simulink model "HighwayLaneChangePlannerTestBench"  (R2024b)
settings: Solver=FixedStepAuto  StartTime=0.0  StopTime=scenario.StopTime  FixedStep=Ts  RelTol=1e-3
PostLoadFcn:
  | helperSLHighwayLaneChangePlannerSetup
values from neighbouring files (symbols this model uses):
  change_difficulty_coeff = 1.0    (= 1)    [helperSLHighwayLaneChangePlannerSetup.m]
  degree = 5    [HelperLCPlannerDefaultData.m]    (also in helperSLHighwayLaneChangePlannerSetup.m)
  egoInitialPose = evalin('base','egoInitialPose')    [HelperPlotLCPlannerStatus.m]    (also in helperSLHighwayLaneChangePlannerSetup.m = struct('ActorID', EgoActor.ActorID,                         )
  lane_change_coeff = 1.0    (= 1)    [helperSLHighwayLaneChangePlannerSetup.m]
  lane_keeping_coeff = 1.0    (= 1)    [helperSLHighwayLaneChangePlannerSetup.m]
  lane_width_coeff = 0.25    [helperSLHighwayLaneChangePlannerSetup.m]
  mapInfo = struct('NumLanes', numLanes,'LaneWidth', zeros(maxNumLanes,1),                  'LaneCenters', zeros(maxNumLanes,1),'NumGlobalPlanPoints',                  size(globalPlanPoints,1), 'GlobalPlanPoints',                  zeros(maxGlobalPlanPoints,2), 'LaneLateralBoundary', zeros(maxNumLanes, 2))    [helperSLHighwayLaneChangePlannerSetup.m]
  MaxFront = 20    [helperSLHighwayLaneChangePlannerSetup.m]
  MaxRear = 20    [helperSLHighwayLaneChangePlannerSetup.m]
  MaxTTC = 5    [helperSLHighwayLaneChangePlannerSetup.m]
  MinTTC = 3    [helperSLHighwayLaneChangePlannerSetup.m]
  num_piece = timeHorizon / 0.5    (= 8)    [helperSLHighwayLaneChangePlannerSetup.m]
  planningResolution = 0.5    [helperSLHighwayLaneChangePlannerSetup.m]
  timeHorizon = 4    [helperSLHighwayLaneChangePlannerSetup.m]
  timeResolution = 0.1    [helperSLHighwayLaneChangePlannerSetup.m]
  Useresample = true    [helperSLHighwayLaneChangePlannerSetup.m]
undefined symbols (not defined in the file or in its folder): actorProfiles, assessment, egoActorID, Feasible_coeff, maxLatAccel, maxLatVelocity, maxLonAccel, maxLonVelocity, minLatVelocity, minLonVelocity, Ts
libraries: simulink x7, drivingscenarioandsensors x2
settings Model: Creator=The MathWorks, Inc.  LastModifiedBy=grape4314
settings SolverCC: ZeroCrossAlgorithm=Adaptive  AlgebraicLoopSolver=TrustRegion  MaxZcPerStep=1
settings DataIOCC: SaveOutput=off  ReturnWorkspaceOutputs=off
settings OptimizationCC: ReuseModelBlockBuffer=off  ZeroExternalMemoryAtStartup=off  ZeroInternalMemoryAtStartup=off  OptimizeBlockOrder=speed
settings DebuggingCC: MaskedZcDiagnostic=none  IgnoredZcDiagnostic=none  UnconnectedInputMsg=warning  UnconnectedOutputMsg=warning  UnconnectedLineMsg=warning  SubsystemReferenceDiagnosticForUnitTest=warning
settings ModelReferenceCC: EnableRefExpFcnMdlSchedulingChecks=on
settings RTWCC: Description=Embedded Coder  SystemTargetFile=ert.tlc  TemplateMakefile=ert_default_tmf  PortableWordSizes=on  CodeProfilingSaveOptions=AllData  TargetLang=C++  GPUComputeCapability=3.5  DLArmComputeVersion=19.05
settings CodeAppCC: ForceParamTrailComments=on  IgnoreCustomStorageClasses=off  OperatorAnnotations=on  SimulinkDataObjDesc=on  SFDataObjDesc=on  InsertBlockDesc=on
settings ERTTargetCC: TargetLangStandard=C++03 (ISO)  GenerateSampleERTMain=on  CodeInterfacePackaging=C++ class  InlinedParameterPlacement=Hierarchical  RootIOFormat=Structure reference  ERTCustomFileTemplate=example_file_process.tlc  DynamicArrayContainerType=coder::array
settings ConfigComp: CovScope=ReferencedModels  CovIncludeTopModel=off  CovMetricSettings=dtrzoibwe

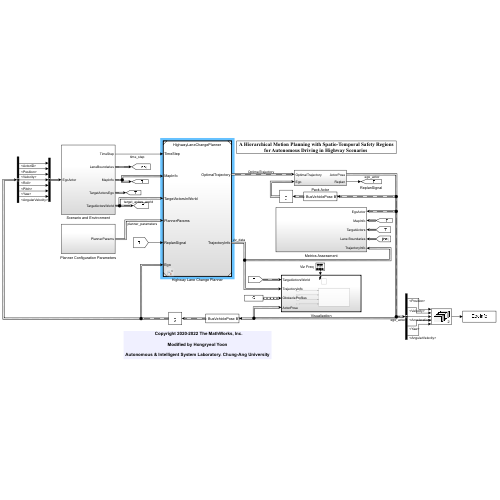
[thumbnail: Simulink's stored preview of the top-level diagram]
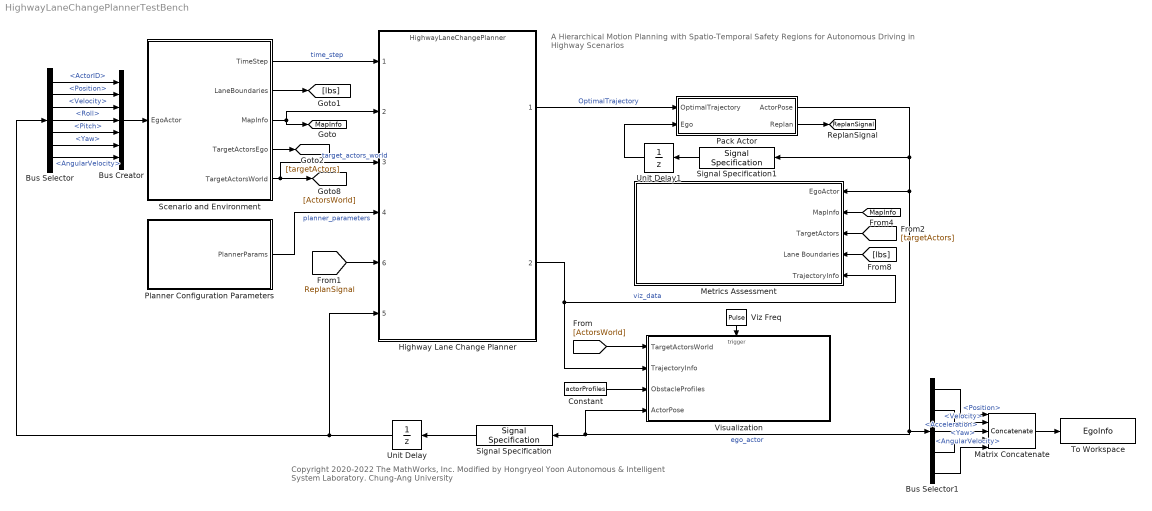
== system HighwayLaneChangePlannerTestBench ==
  note: A Hierarchical Motion Planning with Spatio-Temporal Safety Regions for Autonomous Driving in Highway Scenarios
  note: Copyright 2020-2022 The MathWorks, Inc.
      |
      | Modified by Hongryeol Yoon
      |
      | Autonomous & Intelligent System Laboratory. Chung-Ang University
  Bus Creator : BusCreator  Inputs=7  OutDataTypeStr=Bus: BusVehiclePoseNoAccel
  Bus Selector : BusSelector  OutputSignals=ActorID,Position,Velocity,Roll,Pitch,Yaw,AngularVelocity
  Bus Selector1 : BusSelector  OutputSignals=Position,Velocity,Acceleration,Yaw,AngularVelocity
  Constant : Constant  Value=actorProfiles  OutDataTypeStr=Bus: BusActorProfiles
  Highway Lane Change Planner : ModelReference  ModelNameDialog=HighwayLaneChangePlanner.slx  SimulationMode=Normal  ModelReferenceVersion=10.890
      settings: PortSchema="{\"entries\":[{\"content\":{\"sides\":[{\"content\":{\"connectorIds\":[\"In1\",\"In2\",\"In3\",\"In4\",\"In6\",\"In5\"]},\"type\":\"ConnectorPlacement.EquallySpacedRectSide\",\"uuid\":\"8044d8bb-367a-43f8-b195-4991807fb404\"},{\"content\":{\"connectorIds\":[\"Out1\",\"Out2\"],\"side\":\"RIGHT\"},\"type\":\"ConnectorPlacement.EquallySpacedRectSide\",\"uuid\":\"ee3faf87-dd00-4278-a4db-064b7bf25d12\"},{\"content\":{\"side\":\"TOP\"},\"type\":\"ConnectorPlacement.EquallySpacedRectSide\",\"uuid\":\"9b87e704-685c-45b5-ad58-dd02a7899d78\"}]},\"type\":\"ConnectorPlacement.EquallySpacedConnector\",\"uuid\":\"dfca5ff9-33c4-4b77-827b-e14b0071599c\"}],\"packageUris\":[\"http://schema.mathworks.com/mf0/Connector/R2020b\"],\"version\":\"1.0\"}"
  Matrix Concatenate : Concatenate  NumInputs=5  Mode=Multidimensional array  ConcatenateDimension=2
  Metrics Assessment : Subsystem
  Pack Actor : Subsystem
  Planner Configuration Parameters : Subsystem
  Scenario and Environment : Subsystem
  Signal Specification : SignalSpecification  OutDataTypeStr=Bus: BusVehiclePose  BusOutputAsStruct=on
  Signal Specification1 : SignalSpecification  OutDataTypeStr=Bus: BusVehiclePose  BusOutputAsStruct=on
  To Workspace : ToWorkspace  VariableName=EgoInfo  SaveFormat=Structure With Time  SampleTime=-1
  Unit Delay : UnitDelay  InitialCondition=egoInitialPose  SampleTime=-1  HasFrameUpgradeWarning=on
  Unit Delay1 : UnitDelay  InitialCondition=egoInitialPose  SampleTime=-1  HasFrameUpgradeWarning=on
  Visualization : Subsystem
  Viz Freq : DiscretePulseGenerator  SampleTime=Ts
  tag scope: MapInfo=global, ReplanSignal=global
  wires:
  Scenario and Environment/4(TargetActorsEgo) -> [targetActors]
  Scenario and Environment/2(LaneBoundaries) -> [lbs]
  Highway Lane Change Planner/1 -> Pack Actor/1(OptimalTrajectory)  "OptimalTrajectory"
  Unit Delay/1 -> Bus Selector/1, Highway Lane Change Planner/5
  Signal Specification/1 -> Unit Delay/1
  Scenario and Environment/5(TargetActorsWorld) -> Highway Lane Change Planner/3, [ActorsWorld]  "target_actors_world"
  Scenario and Environment/3(MapInfo) -> Highway Lane Change Planner/2, [MapInfo]
  Constant/1 -> Visualization/3(ObstacleProfiles)
  [ActorsWorld] -> Visualization/1(TargetActorsWorld)
  Planner Configuration Parameters/1(PlannerParams) -> Highway Lane Change Planner/4  "planner_parameters"
  Pack Actor/1(ActorPose) -> Signal Specification1/1, Metrics Assessment/1(EgoActor), Visualization/4(ActorPose), Signal Specification/1, Bus Selector1/1  "ego_actor"
  Highway Lane Change Planner/2 -> Visualization/2(TrajectoryInfo), Metrics Assessment/5(TrajectoryInfo)  "viz_data"
  Scenario and Environment/1(TimeStep) -> Highway Lane Change Planner/1  "time_step"
  [targetActors] -> Metrics Assessment/3(TargetActors)
  [lbs] -> Metrics Assessment/4(Lane Boundaries)
  [MapInfo] -> Metrics Assessment/2(MapInfo)
  Bus Selector/1 -> Bus Creator/1  "<ActorID>"
  Bus Selector/2 -> Bus Creator/2  "<Position>"
  Bus Selector/4 -> Bus Creator/4  "<Roll>"
  Bus Selector/6 -> Bus Creator/6  "<Yaw>"
  Bus Creator/1 -> Scenario and Environment/1(EgoActor)
  Bus Selector/5 -> Bus Creator/5  "<Pitch>"
  Bus Selector/3 -> Bus Creator/3  "<Velocity>"
  Bus Selector/7 -> Bus Creator/7  "<AngularVelocity>"
  Signal Specification1/1 -> Unit Delay1/1
  Unit Delay1/1 -> Pack Actor/2(Ego)
  Pack Actor/2(Replan) -> [ReplanSignal]
  [ReplanSignal] -> Highway Lane Change Planner/6
  Viz Freq/1 -> Visualization/Trigger
  Matrix Concatenate/1 -> To Workspace/1
  Bus Selector1/1 -> Matrix Concatenate/1  "<Position>"
  Bus Selector1/2 -> Matrix Concatenate/2  "<Velocity>"
  Bus Selector1/3 -> Matrix Concatenate/3  "<Acceleration>"
  Bus Selector1/4 -> Matrix Concatenate/4  "<Yaw>"
  Bus Selector1/5 -> Matrix Concatenate/5  "<AngularVelocity>"

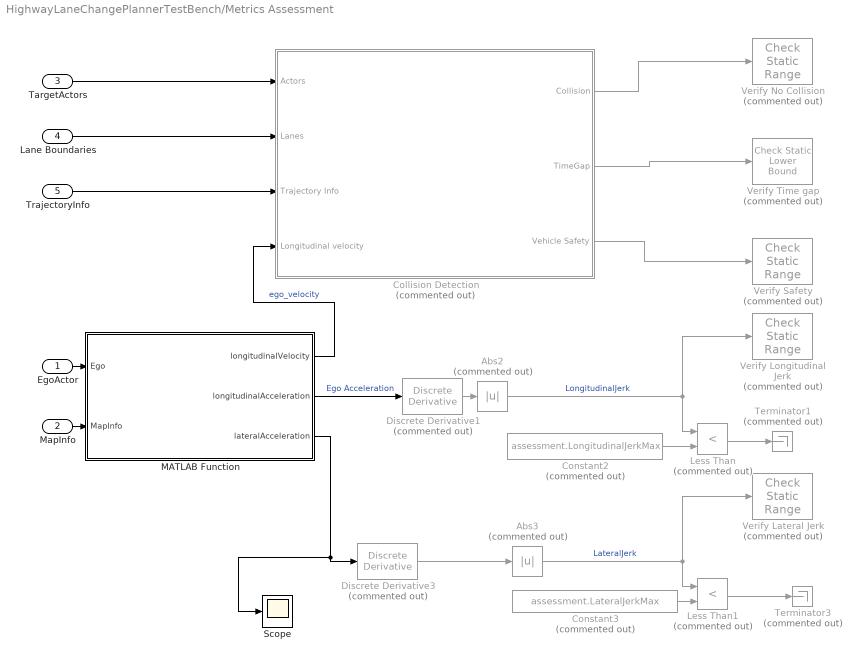
== system HighwayLaneChangePlannerTestBench/Metrics Assessment ==
  EgoActor : Inport
  MapInfo : Inport  Port=2
  TargetActors : Inport  Port=3
  Lane Boundaries : Inport  Port=4
  TrajectoryInfo : Inport  Port=5
  Abs2 : Abs  Commented=on  ZeroCross=off  SaturateOnIntegerOverflow=off
  Abs3 : Abs  Commented=on  ZeroCross=off  SaturateOnIntegerOverflow=off
  Collision Detection : Subsystem  Commented=on
  Constant2 : Constant  Commented=on  Value=assessment.LongitudinalJerkMax
  Constant3 : Constant  Commented=on  Value=assessment.LateralJerkMax
  Discrete Derivative1 : simulink/Discrete/Discrete Derivative  Commented=on  gainval=0.1  ICPrevScaledInput=0.1/Ts  OutMin=[]  OutMax=[]  OutDataType=fixdt(1, 16)  OutScaling=2^-10  DoSatur=off
  Discrete Derivative3 : simulink/Discrete/Discrete Derivative  Commented=on  gainval=0.1  ICPrevScaledInput=0.1/Ts  OutMin=[]  OutMax=[]  OutDataType=fixdt(1, 16)  OutScaling=2^-10  DoSatur=off
  Less Than : RelationalOperator  Commented=on  Operator=<  OutDataTypeStr=boolean  RndMeth=Simplest  InputSameDT=off
  Less Than1 : RelationalOperator  Commented=on  Operator=<  OutDataTypeStr=boolean  RndMeth=Simplest  InputSameDT=off
  MATLAB Function : MATLAB Function  TreatAsAtomicUnit=on
  Scope : Scope
  Terminator1 : Terminator  Commented=on
  Terminator3 : Terminator  Commented=on
  Verify Lateral Jerk : simulink/Model Verification/Check  Static Range  Description=-assessment.LateralJerkMax <= u <= assessment.LateralJerkMax  Commented=on  max=assessment.LateralJerkMax  max_included=on  min=-assessment.LateralJerkMax  min_included=on  enabled=on  stopWhenAssertionFail=off  export=off  icon=graphic
      settings: AttributesFormatString=|
      | ---------------------------------------
      | max = %<max>
      | min = %<min>
  Verify Longitudinal Jerk : simulink/Model Verification/Check  Static Range  Description=-assessment.LongitudinalJerkMax <= u <= assessment.LongitudinalJerkMax  Commented=on  max=assessment.LongitudinalJerkMax  max_included=on  min=-assessment.LongitudinalJerkMax  min_included=on  enabled=on  stopWhenAssertionFail=off  export=off  icon=graphic
      settings: AttributesFormatString=|
      | ---------------------------------------
      | max = %<max>
      | min = %<min>
  Verify No Collision : simulink/Model Verification/Check  Static Range  Description=0 <= u <= 0  Commented=on  max=0  max_included=on  min=0  min_included=on  enabled=on  stopWhenAssertionFail=on  export=off  icon=graphic
  Verify Safety : simulink/Model Verification/Check  Static Range  Description=1 <= u <= 1  Commented=on  max=1  max_included=on  min=1  min_included=on  enabled=on  stopWhenAssertionFail=off  export=off  icon=graphic
  Verify Time gap : simulink/Model Verification/Check Static  Lower Bound  Description=assessment.TimeGap <= u  Commented=on  min=assessment.TimeGap  min_included=on  enabled=on  stopWhenAssertionFail=off  export=off  icon=graphic
      settings: AttributesFormatString=|
      | ---------------------------------------
      | min = %<min>
  wires:
  Collision Detection/1(Collision) -> Verify No Collision/1
  Collision Detection/2(TimeGap) -> Verify Time gap/1
  TrajectoryInfo/1 -> Collision Detection/3(Trajectory Info)
  TargetActors/1 -> Collision Detection/1(Actors)
  Collision Detection/3(Vehicle Safety) -> Verify Safety/1
  Lane Boundaries/1 -> Collision Detection/2(Lanes)
  Discrete Derivative1/1 -> Abs2/1
  Discrete Derivative3/1 -> Abs3/1
  Constant3/1 -> Less Than1/2
  Less Than1/1 -> Terminator3/1
  Constant2/1 -> Less Than/2
  Abs2/1 -> Less Than/1, Verify Longitudinal Jerk/1  "LongitudinalJerk"
  Abs3/1 -> Verify Lateral Jerk/1, Less Than1/1  "LateralJerk"
  Less Than/1 -> Terminator1/1
  EgoActor/1 -> MATLAB Function/1(Ego)
  MapInfo/1 -> MATLAB Function/2(MapInfo)
  MATLAB Function/1(longitudinalVelocity) -> Collision Detection/4(Longitudinal velocity)  "ego_velocity"
  MATLAB Function/2(longitudinalAcceleration) -> Discrete Derivative1/1  "Ego Acceleration"
  MATLAB Function/3(lateralAcceleration) -> Scope/1, Discrete Derivative3/1

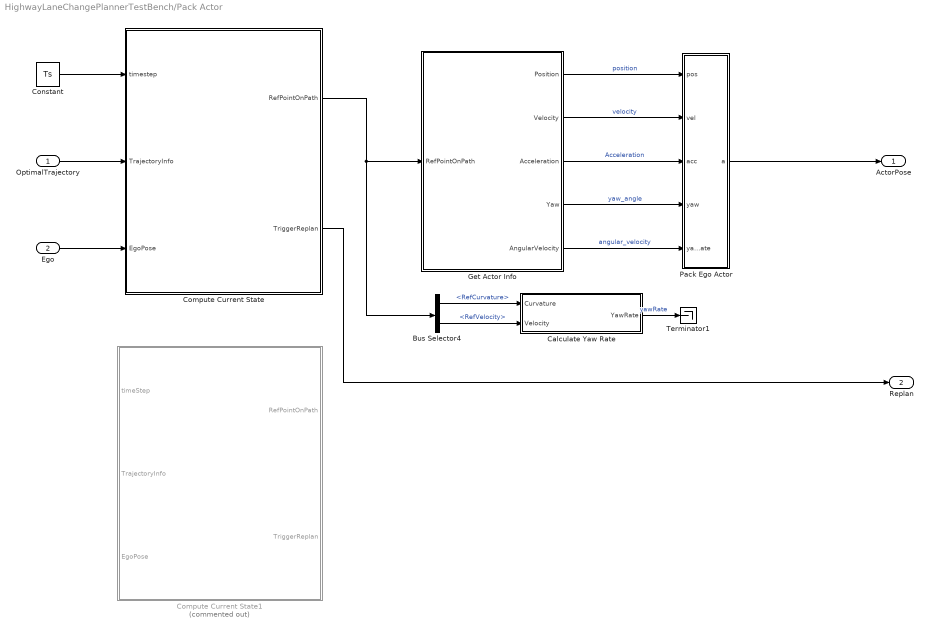
== system HighwayLaneChangePlannerTestBench/Pack Actor ==
  OptimalTrajectory : Inport  SampleTime=Ts
  Ego : Inport  Port=2  OutDataTypeStr=Bus: BusVehiclePose
  Bus Selector4 : BusSelector  OutputSignals=RefCurvature,RefVelocity
  Calculate Yaw Rate : MATLAB Function  TreatAsAtomicUnit=on
  Compute Current State : MATLAB Function  TreatAsAtomicUnit=on
  Compute Current State1 : MATLAB Function  Commented=on  TreatAsAtomicUnit=on
  Constant : Constant  Value=Ts
  Get Actor Info : MATLAB Function  TreatAsAtomicUnit=on
  Pack Ego Actor : MATLAB Function  TreatAsAtomicUnit=on  mask{egoActorID=egoActorID}
      mask prompts: egoActorID "Ego Actor ID"
  Terminator1 : Terminator
  ActorPose : Outport  OutDataTypeStr=Bus: BusVehiclePose
  Replan : Outport  Port=2
  wires:
  Bus Selector4/1 -> Calculate Yaw Rate/1(Curvature)  "<RefCurvature>"
  Bus Selector4/2 -> Calculate Yaw Rate/2(Velocity)  "<RefVelocity>"
  Calculate Yaw Rate/1(YawRate) -> Terminator1/1  "yawRate"
  Pack Ego Actor/1(a) -> ActorPose/1
  Get Actor Info/1(Position) -> Pack Ego Actor/1(pos)  "position"
  Get Actor Info/2(Velocity) -> Pack Ego Actor/2(vel)  "velocity"
  Get Actor Info/3(Acceleration) -> Pack Ego Actor/3(acc)  "Acceleration"
  Get Actor Info/4(Yaw) -> Pack Ego Actor/4(yaw)  "yaw_angle"
  Get Actor Info/5(AngularVelocity) -> Pack Ego Actor/5(yawRate)  "angular_velocity"
  OptimalTrajectory/1 -> Compute Current State/2(TrajectoryInfo)
  Constant/1 -> Compute Current State/1(timestep)
  Ego/1 -> Compute Current State/3(EgoPose)
  Compute Current State/1(RefPointOnPath) -> Bus Selector4/1, Get Actor Info/1(RefPointOnPath)
  Compute Current State/2(TriggerReplan) -> Replan/1

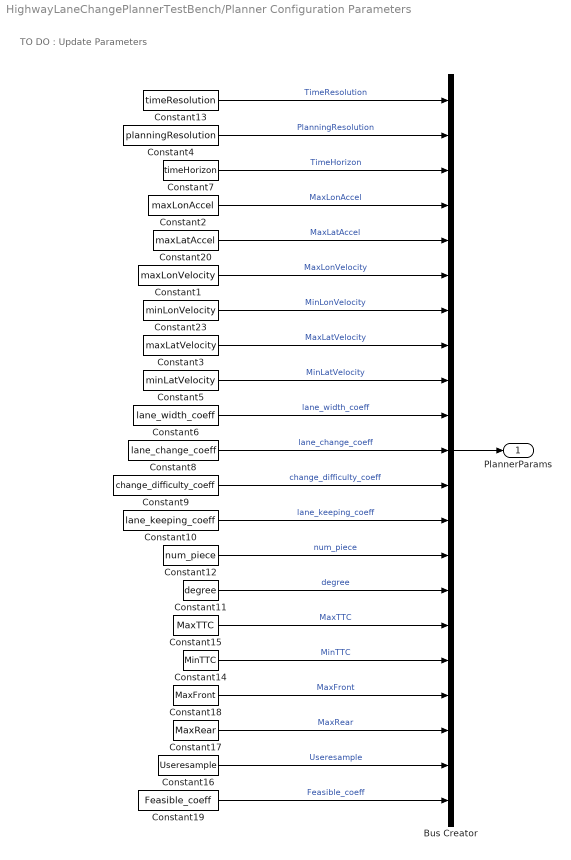
== system HighwayLaneChangePlannerTestBench/Planner Configuration Parameters ==
  note: TO DO : Update Parameters
  Bus Creator : BusCreator  Inputs=21  OutDataTypeStr=Bus: BusPlannerParams  NonVirtualBus=on
  Constant1 : Constant  Value=maxLonVelocity
  Constant10 : Constant  Value=lane_keeping_coeff
  Constant11 : Constant  Value=degree
  Constant12 : Constant  Value=num_piece
  Constant13 : Constant  Value=timeResolution
  Constant14 : Constant  Value=MinTTC
  Constant15 : Constant  Value=MaxTTC
  Constant16 : Constant  Value=Useresample
  Constant17 : Constant  Value=MaxRear
  Constant18 : Constant  Value=MaxFront
  Constant19 : Constant  Value=Feasible_coeff
  Constant2 : Constant  Value=maxLonAccel
  Constant20 : Constant  Value=maxLatAccel
  Constant23 : Constant  Value=minLonVelocity
  Constant3 : Constant  Value=maxLatVelocity
  Constant4 : Constant  Value=planningResolution
  Constant5 : Constant  Value=minLatVelocity
  Constant6 : Constant  Value=lane_width_coeff
  Constant7 : Constant  Value=timeHorizon
  Constant8 : Constant  Value=lane_change_coeff
  Constant9 : Constant  Value=change_difficulty_coeff
  PlannerParams : Outport  OutDataTypeStr=Bus: BusPlannerParams
  wires:
  Constant13/1 -> Bus Creator/1  "TimeResolution"
  Constant1/1 -> Bus Creator/6  "MaxLonVelocity"
  Constant18/1 -> Bus Creator/18  "MaxFront"
  Constant14/1 -> Bus Creator/17  "MinTTC"
  Constant7/1 -> Bus Creator/3  "TimeHorizon"
  Constant3/1 -> Bus Creator/8  "MaxLatVelocity"
  Constant17/1 -> Bus Creator/19  "MaxRear"
  Constant6/1 -> Bus Creator/10  "lane_width_coeff"
  Constant23/1 -> Bus Creator/7  "MinLonVelocity"
  Constant16/1 -> Bus Creator/20  "Useresample"
  Constant9/1 -> Bus Creator/12  "change_difficulty_coeff"
  Constant5/1 -> Bus Creator/9  "MinLatVelocity"
  Constant20/1 -> Bus Creator/5  "MaxLatAccel"
  Constant15/1 -> Bus Creator/16  "MaxTTC"
  Constant8/1 -> Bus Creator/11  "lane_change_coeff"
  Constant4/1 -> Bus Creator/2  "PlanningResolution"
  Constant2/1 -> Bus Creator/4  "MaxLonAccel"
  Constant10/1 -> Bus Creator/13  "lane_keeping_coeff"
  Bus Creator/1 -> PlannerParams/1
  Constant12/1 -> Bus Creator/14  "num_piece"
  Constant11/1 -> Bus Creator/15  "degree"
  Constant19/1 -> Bus Creator/21  "Feasible_coeff"

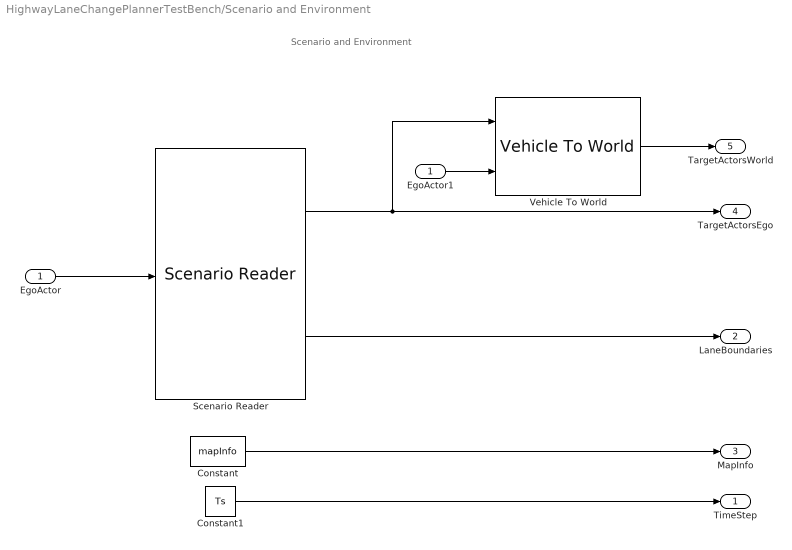
== system HighwayLaneChangePlannerTestBench/Scenario and Environment ==
  note: Scenario and Environment
  EgoActor : Inport
  Constant : Constant  Value=mapInfo  OutDataTypeStr=Bus: BusMapInfo
  Constant1 : Constant  Value=Ts
  EgoActor1 : InportShadow
  Scenario Reader : drivingscenarioandsensors/Scenario Reader  ScenarioSource=From workspace  ScenarioFileName=CurevedRoadNetwork.mat  ScenarioVariableName=scenario  OutputCoordinateSystem=Vehicle coordinates  EgoVehicleSource=Input port  EgoVehicleActorID=egoInitialPose.ActorID  OrientVehiclesOnRoad=off  OutputEgoVehiclePose=off  OutputEgoVehicleState=off  SampleTime=0.1  LaneBoundaryOutput=Ego vehicle lane boundaries  LaneBoundaryDistance=0:0.5:60  LaneBoundaryLocation=Center of lane markings  BusNameSource=Property  BusName=BusActorsEgo  BusNumActorsSource=Scenario  BusNumActors=100  BusName2Source=Auto  BusName2=BusLaneBoundaries  BusNumLaneBoundariesSource=Scenario  BusNumLaneBoundaries=10  BusName3Source=Auto  BusName3=BusEgoActor  BusName4Source=Auto  BusName4=BusEgoState  ShowCoordinateLabels=on  SimulateUsing=Interpreted execution
  Vehicle To World : drivingscenarioandsensors/Vehicle To World  BusNameSource=Auto  BusName=BusVehicleToWorldActors  SimulateUsing=Interpreted execution
  TimeStep : Outport
  LaneBoundaries : Outport  Port=2
  MapInfo : Outport  Port=3  OutDataTypeStr=Bus: BusMapInfo
  TargetActorsEgo : Outport  Port=4  OutDataTypeStr=Bus: BusActorsEgo  VectorParamsAs1DForOutWhenUnconnected=off
  TargetActorsWorld : Outport  Port=5
  wires:
  EgoActor/1 -> Scenario Reader/1
  Scenario Reader/1 -> Vehicle To World/1, TargetActorsEgo/1
  Scenario Reader/2 -> LaneBoundaries/1
  Constant/1 -> MapInfo/1
  EgoActor1/1 -> Vehicle To World/2
  Vehicle To World/1 -> TargetActorsWorld/1
  Constant1/1 -> TimeStep/1

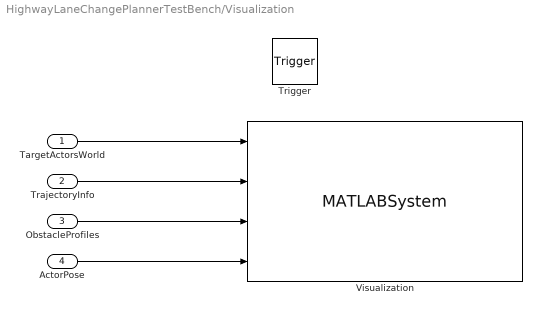
== system HighwayLaneChangePlannerTestBench/Visualization ==
  TargetActorsWorld : Inport
  TrajectoryInfo : Inport  Port=2
  ObstacleProfiles : Inport  Port=3
  ActorPose : Inport  Port=4
  Trigger : TriggerPort  VariantControl=(inherit)  InitialTriggerSignalState=zero  PortDimensions=1
  Visualization : MATLABSystem  System=HelperPlotLCPlannerStatus  EnableTopView=on  EnableTrajTopView=on  EnableChaseView=off  EnableTrajChase=on  EnableCaplistChaseView=on
      mask Type: HelperPlotLCPlannerStatus
      mask Display:
      | disp('HelperPlotLCPlannerStatus');
      | port_label('input',1,'TargetActorsWorld');
      | port_label('input',2,'VisualizationInfo');
      | port_label('input',3,'ObstacleProfiles');
      | port_label('input',4,'EgoActor');
  wires:
  ObstacleProfiles/1 -> Visualization/3
  ActorPose/1 -> Visualization/4
  TrajectoryInfo/1 -> Visualization/2
  TargetActorsWorld/1 -> Visualization/1

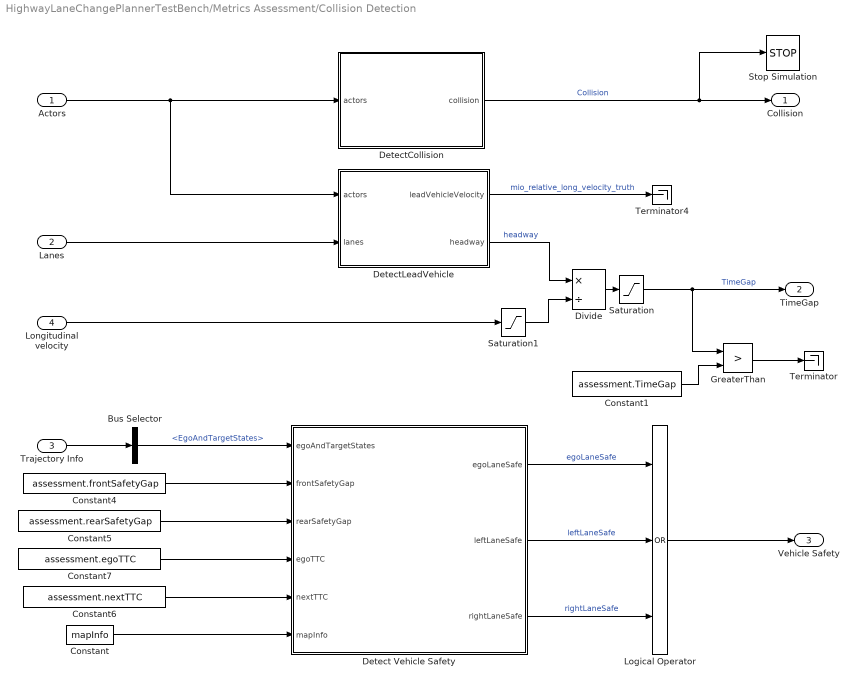
== system HighwayLaneChangePlannerTestBench/Metrics Assessment/Collision Detection ==
  Actors : Inport
  Lanes : Inport  Port=2
  Trajectory Info : Inport  Port=3
  Longitudinal velocity : Inport  Port=4
  Bus Selector : BusSelector  OutputSignals=EgoAndTargetStates
  Constant : Constant  Value=mapInfo  OutDataTypeStr=Bus: BusMapInfo
  Constant1 : Constant  Value=assessment.TimeGap
  Constant4 : Constant  Value=assessment.frontSafetyGap
  Constant5 : Constant  Value=assessment.rearSafetyGap
  Constant6 : Constant  Value=assessment.nextTTC
  Constant7 : Constant  Value=assessment.egoTTC
  Detect Vehicle Safety : MATLAB Function  TreatAsAtomicUnit=on
  DetectCollision : MATLAB Function  TreatAsAtomicUnit=on  mask{actorProfile=actorProfiles, egoActorID=egoInitialPose.ActorID}
      mask prompts: actorProfile "ActorProfiles"
  DetectLeadVehicle : MATLAB Function  TreatAsAtomicUnit=on  mask{vehicleProfiles=actorProfiles}
      mask prompts: vehicleProfiles "Vehicle profiles"
  Divide : Product  Inputs=*/
  GreaterThan : RelationalOperator  Operator=>  OutDataTypeStr=boolean  RndMeth=Simplest  InputSameDT=off
  Logical Operator : Logic  Operator=OR  Inputs=3  AllPortsSameDT=off  OutDataTypeStr=boolean
  Saturation : Saturate  UpperLimit=4  LowerLimit=0
  Saturation1 : Saturate  UpperLimit=100  LowerLimit=0.01
  Stop Simulation : Stop
  Terminator : Terminator
  Terminator4 : Terminator
  Collision : Outport
  TimeGap : Outport  Port=2
  Vehicle Safety : Outport  Port=3
  wires:
  Divide/1 -> Saturation/1
  Actors/1 -> DetectCollision/1(actors), DetectLeadVehicle/1(actors)
  DetectCollision/1(collision) -> Stop Simulation/1, Collision/1  "Collision"
  Saturation1/1 -> Divide/2
  DetectLeadVehicle/2(headway) -> Divide/1  "headway"
  DetectLeadVehicle/1(leadVehicleVelocity) -> Terminator4/1  "mio_relative_long_velocity_truth"
  Saturation/1 -> GreaterThan/1, TimeGap/1  "TimeGap"
  Constant1/1 -> GreaterThan/2
  Lanes/1 -> DetectLeadVehicle/2(lanes)
  GreaterThan/1 -> Terminator/1
  Longitudinal velocity/1 -> Saturation1/1
  Constant6/1 -> Detect Vehicle Safety/5(nextTTC)
  Bus Selector/1 -> Detect Vehicle Safety/1(egoAndTargetStates)  "<EgoAndTargetStates>"
  Constant5/1 -> Detect Vehicle Safety/3(rearSafetyGap)
  Logical Operator/1 -> Vehicle Safety/1
  Constant/1 -> Detect Vehicle Safety/6(mapInfo)
  Constant7/1 -> Detect Vehicle Safety/4(egoTTC)
  Detect Vehicle Safety/3(rightLaneSafe) -> Logical Operator/3  "rightLaneSafe"
  Constant4/1 -> Detect Vehicle Safety/2(frontSafetyGap)
  Detect Vehicle Safety/1(egoLaneSafe) -> Logical Operator/1  "egoLaneSafe"
  Detect Vehicle Safety/2(leftLaneSafe) -> Logical Operator/2  "leftLaneSafe"
  Trajectory Info/1 -> Bus Selector/1

== matlab function HighwayLaneChangePlannerTestBench/Metrics Assessment/Collision Detection/DetectLeadVehicle ==
  data: leadVehicleVelocity output; actors input; headway output; lanes input; vehicleProfiles parameter
function [leadVehicleVelocity, headway]  = detectLeadVehicle(actors, lanes,vehicleProfiles)

% Find the closest vehicle in ego lane
longDist = zeros(1,actors.NumActors);


for i = 1:actors.NumActors
    
    % Positions of the actor with respect to ego in X-direction
    x = actors.Actors(i).Position(1);
    y = actors.Actors(i).Position(2);
    
    % Default longitudinal distance from vehicle
    longDist(i) = inf;
    
    % Check if vehicle is ahead of ego
    if x >= 0
        % Find left lane coordinates closest to vehicle position x
        [~,n] = min(abs(lanes.LaneBoundaries(1).Coordinates(:,1)-x));
        yleftLane = lanes.LaneBoundaries(1).Coordinates(n,2);

        % Find right lane coordinates closest to vehicle position x
        [~,n] = min(abs(lanes.LaneBoundaries(2).Coordinates(:,1)-x));
        yrightLane = lanes.LaneBoundaries(2).Coordinates(n,2);

        % Check if vehicle is in same lane as ego
        if (yrightLane <= y) && (y <= yleftLane)
            longDist(i) = x;
        end       
    end
end
% Minimum distance between vehicle rear axles
[minLongDist,mioIndex] = min(longDist);

% Get lead vehicle information
if isempty(minLongDist) || isinf(minLongDist)
    headway = inf;
    leadVehicleVelocity = inf;
else
    headway = headwayLongDist(minLongDist,mioIndex,vehicleProfiles);
    leadVehicleVelocity = norm(actors.Actors(mioIndex).Velocity);
end

end

function headway = headwayLongDist(dist,mioIndex,vehicleProfiles)
% Longitudinal headway is distance between vehicle rear axles
% reduced by distance of ego rear axle to front and 
% reduced by distance of MIO rear axle to rear

% Notes on origin offset
% - Origin offset is the relative position [x,yz] of vehicle center with 
%   respect to the rear axle
% - Distance rear axle center to vehicle center = negative of origin offset(1)

% Ego distance from rear axle to front
egoProfile = vehicleProfiles(1);
egoDistRearAxleToVehCenter = - egoProfile.OriginOffset(1);
egoDistRearAxleToFront = egoProfile.Length/2 + egoDistRearAxleToVehCenter;

% MIO distance from rear axle to rear
mioProfile = vehicleProfiles(mioIndex);
mioDistRearAxleToVehCenter = - mioProfile.OriginOffset(1);
mioDistRearAxleToRear = mioProfile.Length/2 - mioDistRearAxleToVehCenter;

% Longitudinal headway is distance from front of ego to rear of MIO
headway = dist - egoDistRearAxleToFront - mioDistRearAxleToRear;

end

== matlab function HighwayLaneChangePlannerTestBench/Pack Actor/Pack Ego Actor ==
  data: pos input; a output Bus: BusVehiclePose size=1; vel input; acc input; yaw input; yawRate input; egoActorID parameter
function a = packEgo(pos, vel, acc, yaw, yawRate, egoActorID)
% Pack ego information into a single ego actor bus
%
% Important note:
% Output is a bus of type BusVehiclePose. This bus must match the bus 
% elements expected by Scenario Reader. You can view the 
% bus association using 'Edit Data' in the menu above.

a = struct(...
    'ActorID', egoActorID,...
    'Position', [pos(1) pos(2) 0], ...
    'Velocity', [vel(1) vel(2) 0], ...
    'Acceleration', [acc(1) acc(2) 0], ...
    'Roll', 0, ...
    'Pitch', 0, ...
    'Yaw', yaw, ...
    'AngularVelocity', [0 0 yawRate]);

== matlab function HighwayLaneChangePlannerTestBench/Pack Actor/Calculate Yaw Rate ==
  data: Curvature input; YawRate output; Velocity input
function YawRate = calculateYawRate(Curvature, Velocity)
    YawRate = Curvature.*Velocity;
end

== matlab function HighwayLaneChangePlannerTestBench/Metrics Assessment/MATLAB Function ==
  data: Ego input; longitudinalVelocity output; MapInfo input; longitudinalAcceleration output; lateralAcceleration output
function [longitudinalVelocity, longitudinalAcceleration, lateralAcceleration] = egoFrenetStateConverter(Ego, MapInfo)

persistent RefPathFrenet 
refPath = MapInfo.GlobalPlanPoints(1:MapInfo.NumGlobalPlanPoints,:);
if isempty(RefPathFrenet)    
    RefPathFrenet = referencePathFrenet(refPath);   
else
    %Check for a change in the reference path
    if ~isequal(RefPathFrenet.Waypoints, refPath) 
        refPathNew = referencePathFrenet(refPath);
        RefPathFrenet.Waypoints = refPathNew.Waypoints;
    end
end

kappa = deg2rad(Ego.AngularVelocity(3))/norm(Ego.Velocity);
if (isnan(kappa) || isinf(kappa))
    kappa = 0;
end
egoState = [Ego.Position(1:2), deg2rad(Ego.Yaw), kappa, norm(Ego.Velocity(1:2),2), 0]; 

egoFrenetState = global2frenet(RefPathFrenet, egoState); % [S dS ddS L dL ddL]

longitudinalVelocity = egoFrenetState(2);
longitudinalAcceleration = egoFrenetState(3); % ddS/ddt
lateralAcceleration = egoFrenetState(6) * longitudinalAcceleration; % ddL/ddS * ddS/ddt = ddL/ddt
% [S dS ddS L dL ddL], where S is the arc length and L is the perpendicular
% deviation from the direction of the reference path. Derivatives of S are
% relative to time. Derivatives of L are relative to the arc length, S.

== matlab function HighwayLaneChangePlannerTestBench/Pack Actor/Get Actor Info ==
  data: RefPointOnPath input; Position output; Velocity output; Acceleration output; Yaw output; AngularVelocity output
function [Position, Velocity, Acceleration, Yaw, AngularVelocity] = GetActorInfo(RefPointOnPath)
%GetActorInfo function extracts the information required for actor bus
%information.
%
% This function outputs position, velocity, Yaw angle and angular velocity
% of the ego vehicle. This information is used to update the actor bus.

% Get Position vector
Position = [RefPointOnPath.RefPoseRr(1:2) 0];

% Get orientation of the actor
Yaw = RefPointOnPath.RefPoseRr(3);

% Get Velocity vector
velocity = RefPointOnPath.RefVelocity;
Velocity = [velocity*cosd(Yaw) velocity*sind(Yaw) 0];

% Get Acceleration vector
acceleration = RefPointOnPath.RefAccel;
Acceleration = [acceleration*cosd(Yaw) acceleration*sind(Yaw) 0];

% Get Angular velocity
AngularVelocity = RefPointOnPath.RefAngVel;

end

== matlab function HighwayLaneChangePlannerTestBench/Pack Actor/Compute Current State1 ==
  data: timeStep input; TrajectoryInfo input; RefPointOnPath output Bus: BusRefPointOnPath; EgoPose input; TriggerReplan output
function [RefPointOnPath, TriggerReplan]  = computeCurrentState(timeStep, TrajectoryInfo,...
                                            EgoPose)...
%computeCurrentState estimates the next state of the vehicle based on the
%time or current pose of the ego vehicle.
%
% This function block estimate sthe current pose of the ego vehicle based
% on time or based on current ego pose based on the input from
% StateSelector. If the StateSelector is zero it estimates the pose based
% on current pose, otherwise it estimates state based on time.

    persistent replanTime refPosePrev refCurvPrev refVelPrev refAccPrev sectionStartIndexPrev time
    if isempty(replanTime)
        replanTime = 0;
        refPosePrev = zeros(1,3);
        refCurvPrev = 0;
        refVelPrev = 0;
        refAccPrev = 0;
        sectionStartIndexPrev = 0;
        time = 0;
    end
    
    if TrajectoryInfo.IsNew
        replanTime = time;
    end
    
    % Initialize output structure
    RefPointOnPath = HelperLCPlannerDefaultData.RefPointOnPath;
    
    optimalTrajIndex = TrajectoryInfo.OptimalTrajectoryIndex;
    optimalTrajectory = TrajectoryInfo.GlobalTrajectory(optimalTrajIndex).Trajectory;
    numTrajPoints = TrajectoryInfo.GlobalTrajectory(optimalTrajIndex).NumTrajPoints;
    times = TrajectoryInfo.GlobalTrajectory(optimalTrajIndex).Times;
    
    % Select state based on current pose
    currentPose = [EgoPose.Position(1:2) EgoPose.Yaw];
    [~, refPoses,...
    refCurva, refVelo,...
    refAcc, refAngVel,...
    refCurvDer]  = helperConvertToFixedHorizon(TrajectoryInfo.IsNew,...
                                               numTrajPoints,...
                                               optimalTrajectory, times);
    
    [~,...
    RefPoseRr,...
    RefCurvature,...
    RefVelocity,...
    RefAccel,...
    RefAngVel, RefCurvatureDer,...
    LatOffset,RefYawDiff,...
    sectionStartIndex] = helperComputeCurrentStateBasedOnPose(currentPose,...
                                                              TrajectoryInfo.IsNew,...
                                                              refPoses,...
                                                              refCurva, refVelo,...
                                                              refAcc, refAngVel,...
                                                              refCurvDer,...
                                                              refPosePrev,...
                                                              refCurvPrev,...
                                                              refVelPrev,...
                                                              refAccPrev,...
                                                              sectionStartIndexPrev);
    
    if sectionStartIndex > numTrajPoints
        TriggerReplan = 1;
    else
        TriggerReplan = 0;
    end
    refPosePrev = RefPoseRr;
    refCurvPrev = RefCurvature;
    refVelPrev = RefVelocity;
    refAccPrev = RefAccel;
    sectionStartIndexPrev = sectionStartIndex;                                                 
    
    RefPointOnPath.CurrPoseRr       = [EgoPose.Position(1:2) EgoPose.Yaw];
    RefPointOnPath.RefPoseRr        = RefPoseRr;
    RefPointOnPath.LatOffset        = LatOffset;
    RefPointOnPath.RefCurvature     = RefCurvature;
    RefPointOnPath.RefCurvatureDer  = RefCurvatureDer;
    RefPointOnPath.RefYawDiff       = RefYawDiff;
    RefPointOnPath.RefVelocity      = RefVelocity;
    RefPointOnPath.RefAccel         = RefAccel;
    RefPointOnPath.RefAngVel        = RefAngVel;
    
    time = time + timeStep;
end

== matlab function HighwayLaneChangePlannerTestBench/Metrics Assessment/Collision Detection/Detect Vehicle Safety ==
  data: egoAndTargetStates input; egoLaneSafe output; frontSafetyGap input; rearSafetyGap input; egoTTC input; nextTTC input; mapInfo input; leftLaneSafe output; rightLaneSafe output
function [egoLaneSafe, leftLaneSafe, rightLaneSafe]  = vehicleSafetyDetection(egoAndTargetStates, frontSafetyGap, rearSafetyGap, egoTTC, nextTTC, mapInfo)

egoFrenetState = egoAndTargetStates.EgoFrenetState;

numTargets = egoAndTargetStates.NumTargetActors;
targetFrenetStates = egoAndTargetStates.TargetFrenetStates(1:numTargets, :);

curEgoLane = helperDetectLaneNumber(mapInfo,egoFrenetState(4));

targetLanes = zeros(numTargets,1);
targetTTCs = zeros(numTargets,1);
targetRanges = zeros(numTargets,1);
targetVels = zeros(numTargets,1);
targetFront = zeros(numTargets,1);
mioSafe = zeros(numTargets,1);
% egoLaneSafe = 0;
leftLaneSafe = false;
rightLaneSafe = false;
for i = 1:numTargets
        % Get MIO lane
        targetLanes(i) = helperDetectLaneNumber(mapInfo, targetFrenetStates(i,4));        
        
        % Calculate TTC and other attributes of MIOs with ego vehicle
        [targetRanges(i),~,targetVels(i),targetTTCs(i),targetFront(i)] = helperCalculateTTC(egoFrenetState,targetFrenetStates(i,:));
        mioSafe(i) = checkSafety(targetLanes(i),targetRanges(i),targetTTCs(i),targetFront(i),curEgoLane,frontSafetyGap, rearSafetyGap, egoTTC,nextTTC);        
end

% check ego lane
egoLane = targetLanes==curEgoLane;
% disp(mioSafe(egoLane));
egoLaneSafe = isempty(mioSafe(egoLane)) || all(mioSafe(egoLane));

% check left lane
leftLane = targetLanes==(curEgoLane-1);
if curEgoLane>1
    leftLaneSafe = (isempty(mioSafe(leftLane)) || all(mioSafe(leftLane))); 
end

% check right lane
rightLane = targetLanes==(curEgoLane+1);
if curEgoLane<mapInfo.NumLanes 
    rightLaneSafe = (isempty(mioSafe(rightLane)) || all(mioSafe(rightLane)));
end
end
function isSafe = checkSafety(Lane,Range,TTC,Front,EgoLane,frontSafetyGap,rearSafetyGap,egoTTC,nextTTC)
%checkSafety function checks for safety of current ego lane, and it's
%adjacent lanes.

% default: current lane is unsafe
isSafe = true;

if Front
    SafetyGap = frontSafetyGap;
else
    SafetyGap = rearSafetyGap;
end

if Lane==EgoLane % ego lane
    if Range < SafetyGap || ... % mio is too close?
            (TTC < 0 && ... % mio is approaching
            abs(TTC) < egoTTC) % TTC is too small?
        isSafe = false; % current lane is unsafe
    end
else % left or right lane
    if Range < SafetyGap || ... % mio is too close?
            (TTC < 0 && ... % mio is approaching
            abs(TTC) < nextTTC) % TTC is too small?
        isSafe = false; % current lane is unsafe
    end   
end

end

== matlab function HighwayLaneChangePlannerTestBench/Pack Actor/Compute Current State ==
  data: timestep input; TrajectoryInfo input; EgoPose input; RefPointOnPath output Bus: BusRefPointOnPath; TriggerReplan output
function [RefPointOnPath, TriggerReplan]  = computeCurrentState(timestep, ...
                                                                TrajectoryInfo, ...
                                                                EgoPose)
% computeCurrentState estimates the next state of the vehicle based on the
% time or current pose of the ego vehicle.
%
% This function block estimate sthe current pose of the ego vehicle based
% on time or based on current ego pose based on the input from
% StateSelector. If the StateSelector is zero it estimates the pose based
% on current pose, otherwise it estimates state based on time.

persistent replanTime time prev_new prev_resample
if isempty(replanTime)
    replanTime = 0;
    time = 0;
    prev_new = false;
    prev_resample = false;
end

if (TrajectoryInfo.IsNew && ~prev_new) || (TrajectoryInfo.Isresample && ~prev_resample)
    % Time trigger에 의한 궤적이 생성된 경우,
    % Event trigger에 의해 새로운 궤적이 선택된 경우
    replanTime = time;
end

% Initialize output structure
RefPointOnPath = HelperLCPlannerDefaultData.RefPointOnPath;

optimalTrajIndex = TrajectoryInfo.OptimalTrajectoryIndex;
optimalTrajectory = TrajectoryInfo.GlobalTrajectory(optimalTrajIndex).Trajectory;
numTrajPoints = TrajectoryInfo.GlobalTrajectory(optimalTrajIndex).NumTrajPoints;
times = TrajectoryInfo.GlobalTrajectory(optimalTrajIndex).Times;
durationtime = TrajectoryInfo.GlobalTrajectory(optimalTrajIndex).DurationTime;
resample = TrajectoryInfo.Isresample;

% Check StateSelector
% Select state based on time
[RefPoseRr,  RefCurvature,...
RefVelocity, RefAccel,...
RefAngVel, RefCurvatureDer,...
LatOffset, RefYawDiff,...
TriggerReplan] = helperComputeCurrentStateBasedOnTime(time,...
                                                      replanTime,...
                                                      numTrajPoints,...
                                                      optimalTrajectory,...
                                                      durationtime,...
                                                      resample, ...
                                                      times, ...
                                                      timestep);                                                  

RefPointOnPath.CurrPoseRr       = [EgoPose.Position(1:2) EgoPose.Yaw];
RefPointOnPath.RefPoseRr        = RefPoseRr;
RefPointOnPath.LatOffset        = LatOffset;
RefPointOnPath.RefCurvature     = RefCurvature;
RefPointOnPath.RefCurvatureDer  = RefCurvatureDer;
RefPointOnPath.RefYawDiff       = RefYawDiff;
RefPointOnPath.RefVelocity      = RefVelocity;
RefPointOnPath.RefAccel         = RefAccel;
RefPointOnPath.RefAngVel        = RefAngVel;

time = time + timestep;
prev_new = TrajectoryInfo.IsNew;
prev_resample = resample;
end

== matlab function HighwayLaneChangePlannerTestBench/Metrics Assessment/Collision Detection/DetectCollision ==
  data: actors input; collision output; actorProfile parameter; egoActorID parameter
%% collisionDetect
% Detects if there is any collision while running the model.
function collision  = collisionDetect(actors, actorProfile, egoActorID)
coder.extrinsic('area');
coder.extrinsic('intersect');
coder.extrinsic('union');

egoActor.Position = [0 0];
egoActor.Yaw = 0;
p1 = vehicle2polyshape(egoActor,1.8,4.7,1,[1 0.1]);

collision = false;

overlapRatio = double(0);
actorIdx = 1;
for i = 1:numel(actorProfile)
    if actorProfile(i).ActorID ~= egoActorID
        w = actorProfile(i).Width;
        h = actorProfile(i).Length;
        RO = actorProfile(i).Length * 0.5 + actorProfile(i).OriginOffset(1);
        p2 = vehicle2polyshape(actors.Actors(actorIdx),w,h,RO,[0 0]);
        
        overlapRatio = area(intersect(p1,p2))/area(union(p1,p2));
        
        if overlapRatio > 0.01
            collision = true; % collision detected
            return;
        end
        actorIdx = actorIdx + 1;
    end
end

end

function pshape = vehicle2polyshape(vehicle,w,h,RO,margin)
% vehicle.Position : position (x,y) of vehicle
% vehicle.Yaw : orientation of vehicle
% w: width
% h: height
% RO: read overhang

coder.extrinsic('polyshape');
coder.extrinsic('rotate');

x = vehicle.Position(1);
y = vehicle.Position(2);
theta = vehicle.Yaw - 90;

xcoord = [x-w/2-margin(2), x+w/2+margin(2), x+w/2+margin(2), x-w/2-margin(2)];
ycoord = [y-RO-margin(1), y-RO-margin(1), y+h-RO+margin(1), y+h-RO+margin(1)];
pshape = rotate(polyshape(xcoord, ycoord), theta, [x, y]);
end
